simulink model "Modele_dynamique_direct"  (R2018a)
settings: Solver=VariableStepAuto  StartTime=0.0  StopTime=10.0  RelTol=1e-3
values from neighbouring files (symbols this model uses):
  dq_dt_0 = [0.5; 1.0; -0.5; 0.5; 1.0; -0.5]    [Q17Test.m]    (also in Q20Test.m = zeros(6,1))
  q_0 = qi    [Q17Test.m]    (also in Q20Test.m = q_di)
settings Model: Creator=gabri  LastModifiedBy=gabri

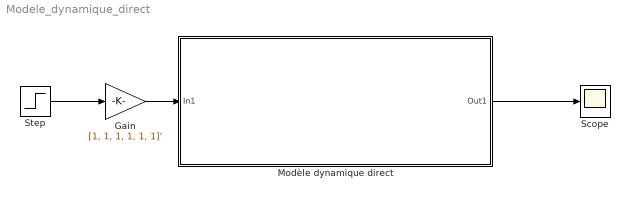
== system Modele_dynamique_direct ==
  Gain : Gain  Gain=[1, 1, 1, 1, 1, 1]'
  Modèle dynamique direct : Subsystem
  Scope : Scope
  Step : Step  SampleTime=0  VectorParams1D=off
  wires:
  Step/1 -> Gain/1
  Modèle dynamique direct/1(Out1) -> Scope/1
  Gain/1 -> Modèle dynamique direct/1(In1)

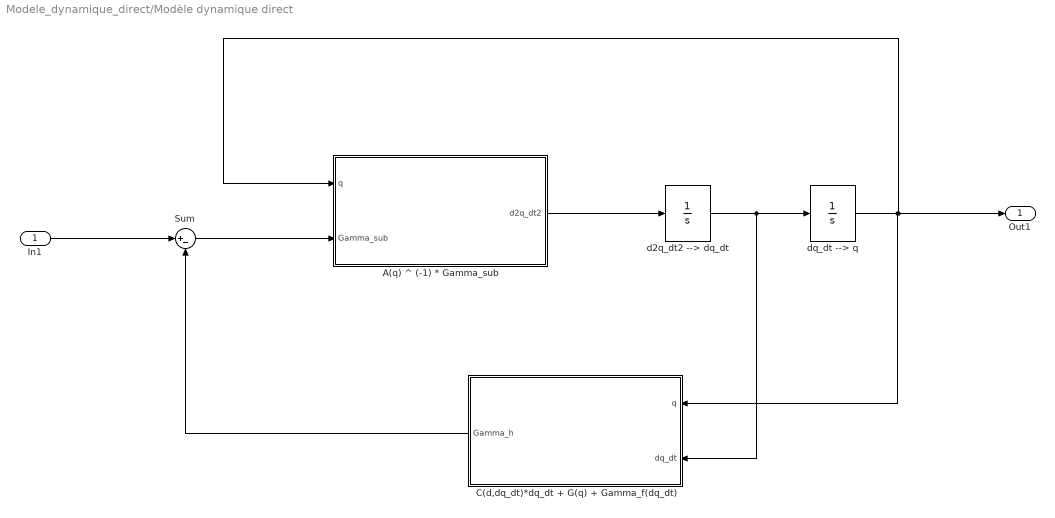
== system Modele_dynamique_direct/Modèle dynamique direct ==
  In1 : Inport
  A(q) ^ (-1) * Gamma_sub : MATLAB Function  TreatAsAtomicUnit=on
  C(d,dq_dt)*dq_dt + G(q) + Gamma_f(dq_dt) : MATLAB Function  TreatAsAtomicUnit=on
  Sum : Sum  Inputs=|+-
  d2q_dt2 --> dq_dt : Integrator  InitialCondition=dq_dt_0
  dq_dt --> q : Integrator  InitialCondition=q_0
  Out1 : Outport
  wires:
  In1/1 -> Sum/1
  d2q_dt2 --> dq_dt/1 -> C(d,dq_dt)*dq_dt + G(q) + Gamma_f(dq_dt)/2(dq_dt), dq_dt --> q/1
  A(q) ^ (-1) * Gamma_sub/1(d2q_dt2) -> d2q_dt2 --> dq_dt/1
  C(d,dq_dt)*dq_dt + G(q) + Gamma_f(dq_dt)/1(Gamma_h) -> Sum/2
  Sum/1 -> A(q) ^ (-1) * Gamma_sub/2(Gamma_sub)
  dq_dt --> q/1 -> Out1/1, A(q) ^ (-1) * Gamma_sub/1(q), C(d,dq_dt)*dq_dt + G(q) + Gamma_f(dq_dt)/1(q)

== matlab function Modele_dynamique_direct/Modèle dynamique direct/C(d,dq_dt)*dq_dt + G(q) + Gamma_f(dq_dt) ==
  data: q input; Gamma_h output; dq_dt input
function Gamma_h = fcn(q, dq_dt)
%%% Gamma_h(q, dq_dt) = C(d,dq_dt)*dq_dt + G(q) + Gamma_f(dq_dt)

C = CalculCoupleCoriolisCentrifuge(q', dq_dt');
C = C';
G = CalculCoupleGravite(q);
Gamma_f = CalculCoupleFrottement(dq_dt);

Gamma_h = C * dq_dt + G + Gamma_f;

end

== matlab function Modele_dynamique_direct/Modèle dynamique direct/A(q) ^ (-1) * Gamma_sub ==
  data: q input; d2q_dt2 output; Gamma_sub input
function d2q_dt2 = fcn(q, Gamma_sub)
%%% d2t_dt2 = A(q)^(-1) * Gamma_sub

A = CalculMatriceInertie(q);

d2q_dt2 = A \ Gamma_sub;

end
